simulink model "ISTR_Discrete_Non_Linear"  (Simulink 9.1)
settings: Solver=ode45  StartTime=0.0  StopTime=15*Tuc  RelTol=1e-3  EnableMultiTasking=on
values from neighbouring files (symbols this model uses):
  a0 = 0    [ISTR_Discrete_Non_Linear_init.m]
  a1 = -1.991    [ISTR_Discrete_Non_Linear_init.m]
  a2 = 0.9968    [ISTR_Discrete_Non_Linear_init.m]
  A_ch1 = pi*(100/2)^2    (= 7853.98163397)    [ISTR_Discrete_Non_Linear_init.m]
  A_ch2 = A_ch1    (= 7853.98163397)    [ISTR_Discrete_Non_Linear_init.m]
  A_p = pi*(d/2)^2    (= 78.5398163397)    [ISTR_Discrete_Non_Linear_init.m]
  am1 = -1.888    [ISTR_Discrete_Non_Linear_init.m]
  am2 = 0.894    [ISTR_Discrete_Non_Linear_init.m]
  b = 0.21    [ISTR_Discrete_Non_Linear_init.m]
  b0 = 1.247    [ISTR_Discrete_Non_Linear_init.m]
  b1 = 1.245    [ISTR_Discrete_Non_Linear_init.m]
  bm0 = 1+am1+am2    (= 0.006)    [ISTR_Discrete_Non_Linear_init.m]
  C = 0.45*10^-3    (= 0.00045)    [ISTR_Discrete_Non_Linear_init.m]
  d = 10    [ISTR_Discrete_Non_Linear_init.m]
  Gamma = 1.41    [ISTR_Discrete_Non_Linear_init.m]
  h0_1 = 150    [ISTR_Discrete_Non_Linear_init.m]
  h0_2 = h0_1    (= 150)    [ISTR_Discrete_Non_Linear_init.m]
  h1_init = h0_1/2    (= 75)    [ISTR_Discrete_Non_Linear_init.m]
  h2_init = h0_2/2    (= 75)    [ISTR_Discrete_Non_Linear_init.m]
  l = 1000    [ISTR_Discrete_Non_Linear_init.m]
  lambda = 0.95    [ISTR_Discrete_Non_Linear_init.m]
  mu = 10^-3*10^-5    (= 1e-08)    [ISTR_Discrete_Non_Linear_init.m]
  P2_init = 1.0    (= 1)    [ISTR_Discrete_Non_Linear_init.m]
  P_atm = 1    [ISTR_Discrete_Non_Linear_init.m]
  P_init = 1*eye(4,4)    [ISTR_Discrete_Non_Linear_init.m]
  Ps = 1.2    [ISTR_Discrete_Non_Linear_init.m]
  Q_amp = 30    [ISTR_Discrete_Non_Linear_init.m]
  R = 287*10^4    (= 2870000)    [ISTR_Discrete_Non_Linear_init.m]
  Roh_air = 1.2    [ISTR_Discrete_Non_Linear_init.m]
  Roh_w = 998    [ISTR_Discrete_Non_Linear_init.m]
  T0 = 273+20    (= 293)    [ISTR_Discrete_Non_Linear_init.m]
  T1 = 273+20    (= 293)    [ISTR_Discrete_Non_Linear_init.m]
  T2 = T1    (= 293)    [ISTR_Discrete_Non_Linear_init.m]
  Tf = 273+20    (= 293)    [ISTR_Discrete_Non_Linear_init.m]
  theta_init = theta_linear    [ISTR_Discrete_Non_Linear_init.m]
  Ts = 273+20    (= 293)    [ISTR_Discrete_Non_Linear_init.m]
  Tsamp = 1/100    (= 0.01)    [ISTR_Discrete_Non_Linear_init.m]
  Tuc = 3    [ISTR_Discrete_Non_Linear_init.m]
  Wn = 8    [ISTR_Discrete_Non_Linear_init.m]
  zetta = 0.7    [ISTR_Discrete_Non_Linear_init.m]
libraries: commnoisgen2 x1
settings Model: Creator=gshaver  LastModifiedBy=Ahmad
settings DataIOCC: LimitDataPoints=on  SignalLoggingSaveFormat=ModelDataLogs
settings OptimizationCC: ExpressionDepthLimit=2147483647
settings DebuggingCC: SolverPrmCheckMsg=warning  FcnCallInpInsideContextMsg=warning  StateNameClashWarn=warning
settings GRTTargetCC: GeneratePreprocessorConditionals=Disable all

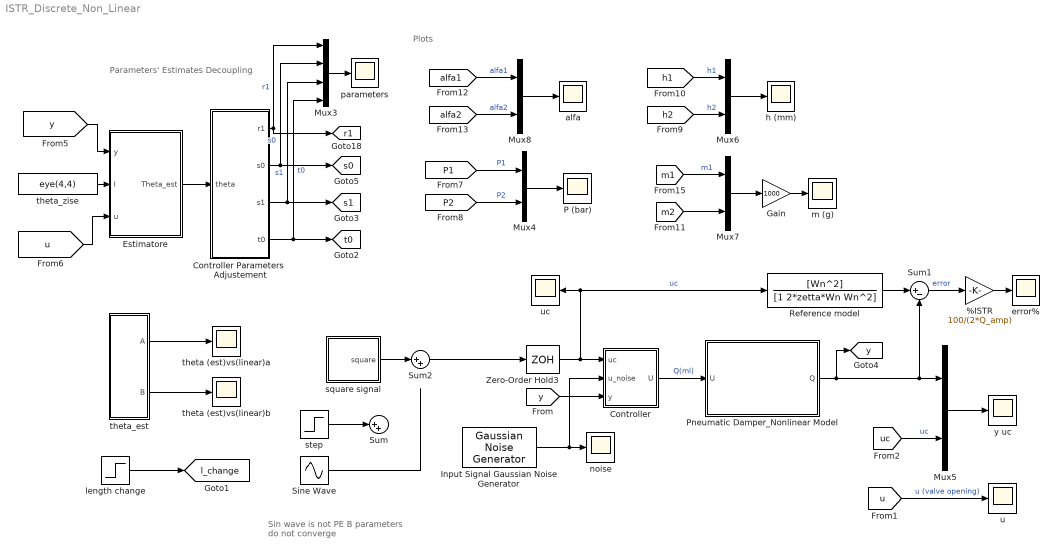
== system ISTR_Discrete_Non_Linear ==
  note: Plots
  note: Sin wave is not PE
      | B parameters do not converge
  note: Parameters' Estimates Decoupling
  %ISTR : Gain  Gain=100/(2*Q_amp)
  Controller : Subsystem
  Controller Parameters  Adjustement : Subsystem
  Estimatore : Subsystem
  Gain : Gain  Gain=1000
  Input Signal Gaussian Noise Generator : commnoisgen2/Gaussian Noise Generator  m=0  d=Noise  s=41  Ts=1/100  frameBased=off  sampPerFrame=1  orient=off  outDataType=double
  Mux3 : Mux
  Mux{4..8} (5 alike) : Mux  Inputs=2
  P (bar) : Scope
  Pneumatic Damper_Nonlinear Model : Subsystem
  Reference model : TransferFcn  Numerator=[Wn^2]  Denominator=[1 2*zetta*Wn Wn^2]
  Sine Wave : Sin  Amplitude=10  Frequency=Tuc  SampleTime=0
  Sum : Sum  Inputs=|++
  Sum1 : Sum  Inputs=|+-
  Sum2 : Sum  Inputs=|++
  Zero-Order Hold3 : ZeroOrderHold  SampleTime=Tsamp
  alfa : Scope
  error% : Scope
  h (mm) : Scope
  length change : Step  Time=0  After=0  SampleTime=0
  m (g) : Scope
  noise : Scope
  parameters : Scope
  square signal : Subsystem
  step : Step  Time=0.01  Before=10  After=0  SampleTime=0
  theta (est)vs(linear)a : Scope
  theta (est)vs(linear)b : Scope
  theta_est : Subsystem
  theta_zise : Constant  Value=eye(4,4)  VectorParams1D=off
  u : Scope
  uc : Scope
  y uc : Scope
  tag scope: l_change=global, r1=global, s0=global, s1=global, t0=global, y=global
  wires:
  [y] -> Estimatore/1(y)
  theta_zise/1 -> Estimatore/2(I)
  [u] -> Estimatore/3(u)
  step/1 -> Sum/1
  Controller Parameters  Adjustement/4("t0 ") -> Mux3/4, [t0]  "t0"
  Controller Parameters  Adjustement/1("r1 ") -> Mux3/1, [r1]  "r1"
  Controller Parameters  Adjustement/2("s0 ") -> Mux3/2, [s0]  "s0"
  Controller Parameters  Adjustement/3("s1 ") -> Mux3/3, [s1]  "s1"
  Sine Wave/1 -> ?
  Controller/1(U) -> Pneumatic Damper_Nonlinear Model/1(U)  "Q(ml)"
  Mux5/1 -> y uc/1
  [u] -> u/1  "u (valve opening)"
  [uc] -> Mux5/2  "uc"
  Estimatore/1(Theta_est) -> Controller Parameters  Adjustement/1(theta)
  Sum1/1 -> %ISTR/1  "error"
  Zero-Order Hold3/1 -> Controller/1(uc), uc/1, Reference model/1  "uc"
  Input Signal Gaussian Noise Generator/1 -> Controller/2(u_noise), noise/1
  length change/1 -> [l_change]
  Mux3/1 -> parameters/1
  [P1] -> Mux4/1  "P1"
  [P2] -> Mux4/2  "P2"
  Mux4/1 -> P (bar)/1
  [h1] -> Mux6/1  "h1"
  [h2] -> Mux6/2  "h2"
  Mux6/1 -> h (mm)/1
  [m1] -> Mux7/1  "m1"
  [m2] -> Mux7/2
  Mux7/1 -> Gain/1
  Gain/1 -> m (g)/1
  [alfa1] -> Mux8/1  "alfa1"
  [alfa2] -> Mux8/2  "alfa2"
  Mux8/1 -> alfa/1
  Reference model/1 -> Sum1/1
  square signal/1(square) -> Sum2/1
  theta_est/1(A) -> theta (est)vs(linear)a/1
  theta_est/2(B) -> theta (est)vs(linear)b/1
  %ISTR/1 -> error%/1
  Sum2/1 -> Zero-Order Hold3/1
  Pneumatic Damper_Nonlinear Model/1("Q  ") -> [y], Mux5/1, Sum1/2
  [y] -> Controller/3(y)

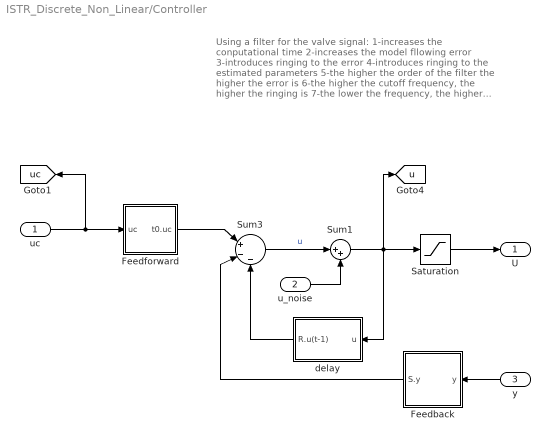
== system ISTR_Discrete_Non_Linear/Controller ==
  note: Using a filter for the valve signal:
      | 1-increases the conputational time
      | 2-increases the model fllowing error
      | 3-introduces ringing to the error
      | 4-introduces ringing to the estimated parameters
      | 5-the higher the order of the filter the higher the error is
      | 6-the higher the cutoff frequency, the higher the ringing is
      | 7-the lower the frequency, the higher the error is
  uc : Inport
  u_noise : Inport  Port=2
  y : Inport  Port=3
  Feedback : Subsystem
  Feedforward : Subsystem
  Saturation : Saturate  UpperLimit=1  LowerLimit=-1
  Sum1 : Sum  Inputs=|++
  Sum3 : Sum  Inputs=|+--
  delay : Subsystem
  U : Outport
  tag scope: u=global, uc=global
  wires:
  uc/1 -> Feedforward/1(uc), [uc]
  Feedforward/1(t0.uc) -> Sum3/1
  Feedback/1(S.y) -> Sum3/2
  delay/1(R.u(t-1)) -> Sum3/3
  Sum3/1 -> Sum1/1  "u"
  u_noise/1 -> Sum1/2
  Sum1/1 -> Saturation/1, [u], delay/1(u)
  Saturation/1 -> U/1
  y/1 -> Feedback/1(y)

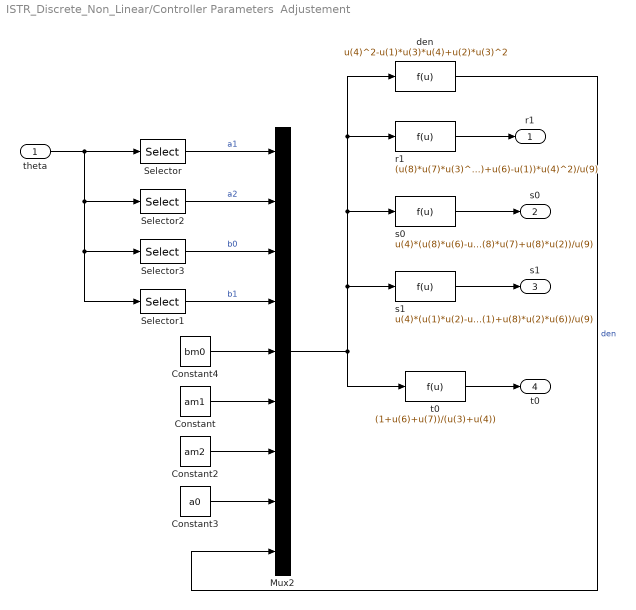
== system ISTR_Discrete_Non_Linear/Controller Parameters  Adjustement ==
  theta : Inport
  Constant : Constant  Value=am1
  Constant2 : Constant  Value=am2
  Constant3 : Constant  Value=a0
  Constant4 : Constant  Value=bm0
  Mux2 : Mux  Inputs=9
  Selector : Selector  NumberOfDimensions=2  InputPortWidth=3  IndexOptions=Index vector (dialog),Index vector (dialog)  Indices=1,1  OutputSizes=1,1
  Selector1 : Selector  NumberOfDimensions=2  InputPortWidth=3  IndexOptions=Index vector (dialog),Index vector (dialog)  Indices=4,1  OutputSizes=1,1
  Selector2 : Selector  NumberOfDimensions=2  InputPortWidth=3  IndexOptions=Index vector (dialog),Index vector (dialog)  Indices=2,1  OutputSizes=1,1
  Selector3 : Selector  NumberOfDimensions=2  InputPortWidth=3  IndexOptions=Index vector (dialog),Index vector (dialog)  Indices=3,1  OutputSizes=1,1
  den : Fcn  Expr=u(4)^2-u(1)*u(3)*u(4)+u(2)*u(3)^2
  r1 : Fcn  Expr=(u(8)*u(7)*u(3)^2+(u(2)-u(7)-u(8)*u(6))*u(3)*u(4)+(u(8)+u(6)-u(1))*u(4)^2)/u(9)
  s0 : Fcn  Expr=u(4)*(u(8)*u(6)-u(2)-u(6)*u(1)+u(1)^2+u(7)-u(1)*u(8))/u(9)+u(3)*(u(6)*u(2)-u(1)*u(2)-u(8)*u(7)+u(8)*u(2))/u(9)
  s1 : Fcn  Expr=u(4)*(u(1)*u(2)-u(6)*u(2)+u(8)*u(7)-u(8)*u(2))/u(9)+u(3)*(u(2)*u(7)-u(2)^2-u(8)*u(7)*u(1)+u(8)*u(2)*u(6))/u(9)
  t0 : Fcn  Expr=(1+u(6)+u(7))/(u(3)+u(4))
  "r1 " : Outport
  "s0 " : Outport  Port=2
  "s1 " : Outport  Port=3
  "t0 " : Outport  Port=4
  wires:
  t0/1 -> "t0 "/1
  s1/1 -> "s1 "/1
  r1/1 -> "r1 "/1
  Mux2/1 -> den/1, r1/1, s0/1, s1/1, t0/1
  s0/1 -> "s0 "/1
  Constant/1 -> Mux2/6
  Selector/1 -> Mux2/1  "a1"
  Constant4/1 -> Mux2/5
  Constant2/1 -> Mux2/7
  Constant3/1 -> Mux2/8
  den/1 -> Mux2/9  "den"
  Selector3/1 -> Mux2/3  "b0"
  theta/1 -> Selector1/1, Selector3/1, Selector2/1, Selector/1
  Selector1/1 -> Mux2/4  "b1"
  Selector2/1 -> Mux2/2  "a2"

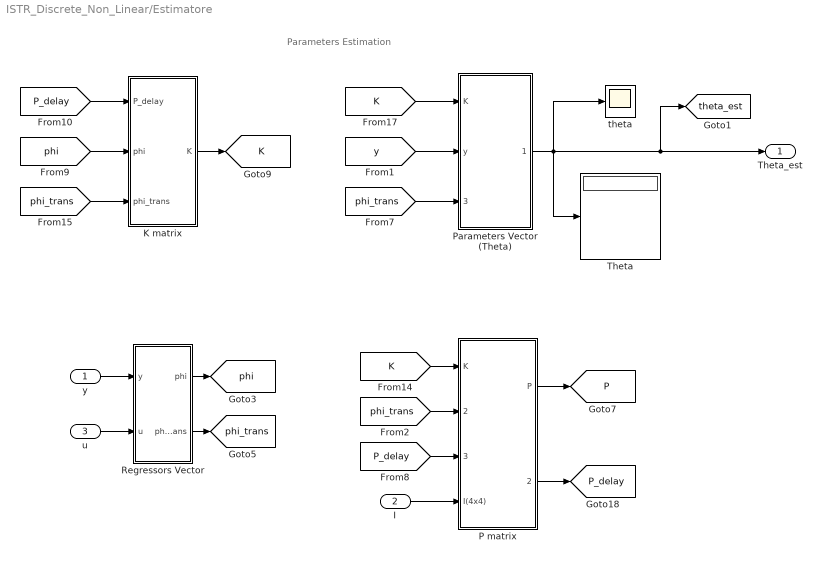
== system ISTR_Discrete_Non_Linear/Estimatore ==
  note: Parameters Estimation
  y : Inport
  I : Inport  Port=2
  u : Inport  Port=3
  K matrix : Subsystem
  P matrix : Subsystem
  Parameters Vector (Theta) : Subsystem
  Regressors Vector : Subsystem
  Theta : Display
  theta : Scope
  Theta_est : Outport
  tag scope: K=global, P=global, P_delay=global, phi=global, phi_trans=global, theta_est=global
  wires:
  [K] -> Parameters Vector (Theta)/1(K)
  y/1 -> Regressors Vector/1(y)
  [phi_trans] -> K matrix/3(phi_trans)
  [phi] -> K matrix/2(phi)
  [P_delay] -> K matrix/1(P_delay)
  K matrix/1(K) -> [K]
  [phi_trans] -> Parameters Vector (Theta)/3(phi_trans)
  Regressors Vector/2(phi_trans) -> [phi_trans]
  u/1 -> Regressors Vector/2(u)
  Regressors Vector/1(phi) -> [phi]
  I/1 -> P matrix/4(I(4x4))
  P matrix/2("P_delay ") -> [P_delay]
  [K] -> P matrix/1(K)
  [phi_trans] -> P matrix/2(phi_trans)
  [P_delay] -> P matrix/3(P_delay)
  P matrix/1(P) -> [P]
  Parameters Vector (Theta)/1(Theta_est) -> theta/1, [theta_est], Theta_est/1, Theta/1
  [y] -> Parameters Vector (Theta)/2(y)

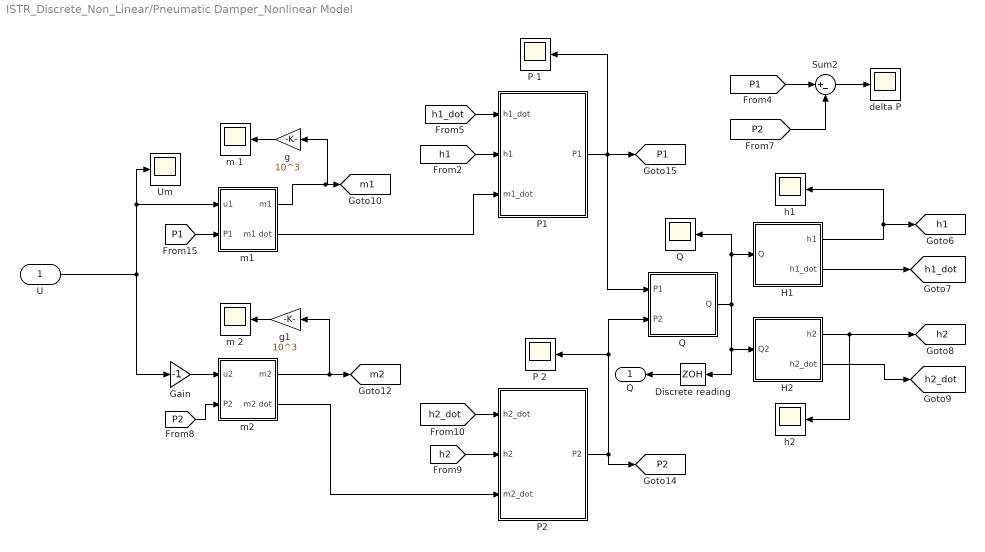
== system ISTR_Discrete_Non_Linear/Pneumatic Damper_Nonlinear Model ==
  U : Inport
  Discrete reading : ZeroOrderHold  SampleTime=Tsamp
  Gain : Gain  Gain=-1
  H1 : Subsystem
  H2 : Subsystem
  P 1 : Scope
  P 2 : Scope
  P1 : Subsystem
  P2 : Subsystem
  Q : Subsystem
  "Q " : Scope
  Sum2 : Sum  Inputs=|+-
  Um : Scope
  delta P : Scope
  g : Gain  Gain=10^3
  g1 : Gain  Gain=10^3
  h1 : Scope
  h2 : Scope
  m 1 : Scope
  m 2 : Scope
  m1 : Subsystem
  m2 : Subsystem
  "Q  " : Outport
  tag scope: P1=global, P2=global, h1=global, h1_dot=global, h2=global, h2_dot=global, m1=global, m2=global
  wires:
  H1/1(h1) -> [h1], h1/1
  H1/2(h1_dot) -> [h1_dot]
  H2/2(h2_dot) -> [h2_dot]
  H2/1(h2) -> h2/1, [h2]
  m1/1(m1) -> g/1, [m1]
  m2/1(m2) -> g1/1, [m2]
  m2/2(m2 dot) -> P2/3(m2_dot)
  [h2_dot] -> P2/1(h2_dot)
  [h1] -> P1/2(h1)
  [h2] -> P2/2(h2)
  P2/1(P2) -> [P2], P 2/1, Q/2(P2)
  U/1 -> Um/1, m1/1(u1), Gain/1
  P1/1(P1) -> P 1/1, Q/1(P1), [P1]
  Gain/1 -> m2/1(u2)
  Q/1(Q) -> Discrete reading/1, H2/1(Q2), H1/1(Q), "Q "/1
  [h1_dot] -> P1/1(h1_dot)
  g/1 -> m 1/1
  [P1] -> Sum2/1
  Sum2/1 -> delta P/1
  [P2] -> Sum2/2
  m1/2(m1 dot) -> P1/3(m1_dot)
  [P2] -> m2/2(P2)
  g1/1 -> m 2/1
  [P1] -> m1/2(P1)
  Discrete reading/1 -> "Q  "/1

== system ISTR_Discrete_Non_Linear/square signal ==
  Pulse Generator1 : DiscretePulseGenerator  PulseType=Time based  Amplitude=-Q_amp  Period=Tuc  PulseWidth=50  PhaseDelay=Tuc/2
  Pulse Generator3 : DiscretePulseGenerator  PulseType=Time based  Amplitude=Q_amp  Period=Tuc  PulseWidth=50
  Sum3 : Sum  Inputs=|++
  square : Outport
  wires:
  Pulse Generator3/1 -> Sum3/1
  Sum3/1 -> square/1
  Pulse Generator1/1 -> Sum3/2

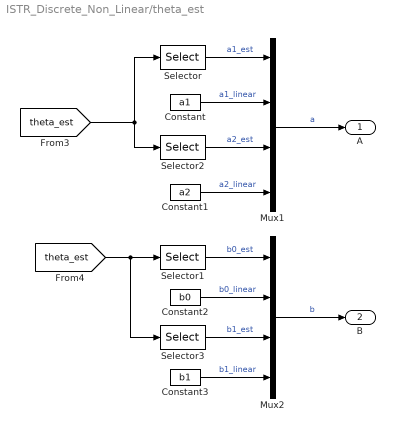
== system ISTR_Discrete_Non_Linear/theta_est ==
  Constant : Constant  Value=a1
  Constant1 : Constant  Value=a2
  Constant2 : Constant  Value=b0
  Constant3 : Constant  Value=b1
  Mux1 : Mux
  Mux2 : Mux
  Selector : Selector  NumberOfDimensions=2  InputPortWidth=3  IndexOptions=Index vector (dialog),Index vector (dialog)  Indices=1,1  OutputSizes=1,1
  Selector1 : Selector  NumberOfDimensions=2  InputPortWidth=3  IndexOptions=Index vector (dialog),Index vector (dialog)  Indices=3,1  OutputSizes=1,1
  Selector2 : Selector  NumberOfDimensions=2  InputPortWidth=3  IndexOptions=Index vector (dialog),Index vector (dialog)  Indices=2,1  OutputSizes=1,1
  Selector3 : Selector  NumberOfDimensions=2  InputPortWidth=3  IndexOptions=Index vector (dialog),Index vector (dialog)  Indices=4,1  OutputSizes=1,1
  A : Outport
  B : Outport  Port=2
  wires:
  Selector2/1 -> Mux1/3  "a2_est"
  Constant3/1 -> Mux2/4  "b1_linear"
  Constant1/1 -> Mux1/4  "a2_linear"
  [theta_est] -> Selector/1, Selector2/1
  Constant2/1 -> Mux2/2  "b0_linear"
  Constant/1 -> Mux1/2  "a1_linear"
  Selector3/1 -> Mux2/3  "b1_est"
  Mux2/1 -> B/1  "b"
  [theta_est] -> Selector1/1, Selector3/1
  Selector/1 -> Mux1/1  "a1_est"
  Mux1/1 -> A/1  "a"
  Selector1/1 -> Mux2/1  "b0_est"

== system ISTR_Discrete_Non_Linear/Controller/Feedback ==
  y : Inport
  Product1 : Product
  Product3 : Product
  Sum4 : Sum  Inputs=|++
  Unit Delay : UnitDelay  SampleTime=-1
  S.y : Outport
  wires:
  y/1 -> Product3/2, Unit Delay/1
  Sum4/1 -> S.y/1
  Product1/1 -> Sum4/2
  Unit Delay/1 -> Product1/1  "y(t-1)"
  Product3/1 -> Sum4/1
  [s1] -> Product1/2
  [s0] -> Product3/1

== system ISTR_Discrete_Non_Linear/Controller/Feedforward ==
  uc : Inport
  Product2 : Product
  t0.uc : Outport
  wires:
  Product2/1 -> t0.uc/1
  [t0] -> Product2/2
  uc/1 -> Product2/1

== system ISTR_Discrete_Non_Linear/Controller/delay ==
  u : Inport
  Product4 : Product
  Unit Delay1 : UnitDelay  SampleTime=-1
  R.u(t-1) : Outport
  wires:
  u/1 -> Unit Delay1/1
  Unit Delay1/1 -> Product4/2  "u(t-1)"
  Product4/1 -> R.u(t-1)/1
  [r1] -> Product4/1

== system ISTR_Discrete_Non_Linear/Estimatore/K matrix ==
  P_delay : Inport
  phi : Inport  Port=2
  phi_trans : Inport  Port=3
  Lambda2 : Constant  Value=lambda  VectorParams1D=off
  Matrix Multiply2 : Product  Multiplication=Matrix(*)
  Matrix Multiply6 : Product  Inputs=***  Multiplication=Matrix(*)
  Matrix Multiply7 : Product  Inputs=/  Multiplication=Matrix(*)
  Matrix Multiply9 : Product  Inputs=**  Multiplication=Matrix(*)
  Sum4 : Sum  Inputs=|++
  K : Outport
  wires:
  Matrix Multiply9/1 -> K/1
  Matrix Multiply7/1 -> Matrix Multiply9/2
  Matrix Multiply2/1 -> Matrix Multiply9/1
  P_delay/1 -> Matrix Multiply6/2, Matrix Multiply2/1
  Lambda2/1 -> Sum4/2
  Matrix Multiply6/1 -> Sum4/1
  Sum4/1 -> Matrix Multiply7/1
  phi_trans/1 -> Matrix Multiply6/1
  phi/1 -> Matrix Multiply6/3, Matrix Multiply2/2

== system ISTR_Discrete_Non_Linear/Estimatore/P matrix ==
  K : Inport
  phi_trans : Inport  Port=2
  P_delay : Inport  Port=3
  I(4x4) : Inport  Port=4
  Gain : Gain  Gain=1/lambda
  Matrix Multiply5 : Product  Multiplication=Matrix(*)
  Matrix Multiply8 : Product  Multiplication=Matrix(*)
  Sum5 : Sum  Inputs=|-+
  Unit Delay6 : UnitDelay  InitialCondition=P_init  SampleTime=Tsamp
  P : Outport
  "P_delay " : Outport  Port=2
  wires:
  phi_trans/1 -> Matrix Multiply8/2
  Matrix Multiply8/1 -> Sum5/1
  K/1 -> Matrix Multiply8/1
  Sum5/1 -> Matrix Multiply5/1
  P_delay/1 -> Matrix Multiply5/2
  Matrix Multiply5/1 -> Gain/1
  Gain/1 -> P/1, Unit Delay6/1
  Unit Delay6/1 -> "P_delay "/1
  I(4x4)/1 -> Sum5/2

== system ISTR_Discrete_Non_Linear/Estimatore/Parameters Vector (Theta) ==
  K : Inport
  y : Inport  Port=2
  phi_trans : Inport  Port=3
  K17 : Scope
  Matrix Multiply3 : Product  Multiplication=Matrix(*)
  Matrix Multiply4 : Product  Multiplication=Matrix(*)
  Sum1 : Sum  Inputs=|+-
  Sum3 : Sum  Inputs=|++
  Unit Delay1 : UnitDelay  InitialCondition=theta_init  SampleTime=Tsamp
  Theta_est : Outport
  wires:
  K/1 -> Matrix Multiply4/1, K17/1
  Matrix Multiply3/1 -> Sum1/2
  phi_trans/1 -> Matrix Multiply3/1
  Unit Delay1/1 -> Sum3/2, Matrix Multiply3/2  "theta(t-1)"
  Sum1/1 -> Matrix Multiply4/2  "theta"
  Matrix Multiply4/1 -> Sum3/1
  Sum3/1 -> Theta_est/1, Unit Delay1/1
  y/1 -> Sum1/1

== system ISTR_Discrete_Non_Linear/Estimatore/Regressors Vector ==
  y : Inport
  u : Inport  Port=2
  Gain : Gain  Gain=-1
  Regressors : Scope
  Transpose : Math  Operator=transpose  SaturateOnIntegerOverflow=on
  Unit Delay1 : UnitDelay  SampleTime=Tsamp
  Unit Delay2 : UnitDelay  SampleTime=Tsamp
  Unit Delay3 : UnitDelay  InitialCondition=0.1  SampleTime=Tsamp
  Unit Delay6 : UnitDelay  SampleTime=Tsamp
  Vector Concatenate : Concatenate  NumInputs=4  Mode=Multidimensional array
  phi : Outport
  phi_trans : Outport  Port=2
  wires:
  Gain/1 -> Unit Delay1/1
  u/1 -> Unit Delay6/1
  Vector Concatenate/1 -> phi/1, Regressors/1, Transpose/1
  y/1 -> Gain/1
  Unit Delay2/1 -> Vector Concatenate/2
  Transpose/1 -> phi_trans/1
  Unit Delay3/1 -> Vector Concatenate/4
  Unit Delay1/1 -> Unit Delay2/1, Vector Concatenate/1
  Unit Delay6/1 -> Vector Concatenate/3, Unit Delay3/1

== system ISTR_Discrete_Non_Linear/Pneumatic Damper_Nonlinear Model/H1 ==
  Q : Inport
  Constant : Constant  Value=A_ch1
  Divide : Product  Inputs=*/
  Integrator : Integrator  InitialCondition=h1_init
  cm-mm : Gain  Gain=-10^3
  h1 : Outport
  h1_dot : Outport  Port=2
  wires:
  Q/1 -> Divide/1
  Integrator/1 -> h1/1  "h1"
  cm-mm/1 -> h1_dot/1, Integrator/1  "h1_dot"
  Divide/1 -> cm-mm/1
  Constant/1 -> Divide/2

== system ISTR_Discrete_Non_Linear/Pneumatic Damper_Nonlinear Model/H2 ==
  Q2 : Inport
  A_pressure_chamber2 : Constant  Value=A_ch2
  Divide : Product  Inputs=*/
  Integrator : Integrator  InitialCondition=h2_init
  cm-mm : Gain  Gain=10^3
  h2 : Outport
  h2_dot : Outport  Port=2
  wires:
  A_pressure_chamber2/1 -> Divide/2
  Q2/1 -> Divide/1
  Integrator/1 -> h2/1  "h2"
  Divide/1 -> cm-mm/1  "h2_dot"
  cm-mm/1 -> Integrator/1, h2_dot/1

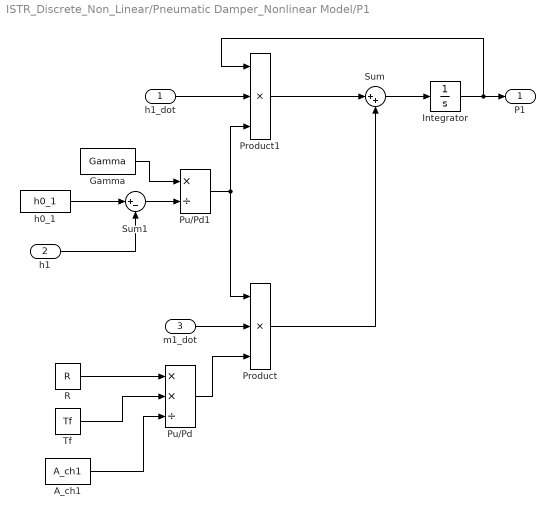
== system ISTR_Discrete_Non_Linear/Pneumatic Damper_Nonlinear Model/P1 ==
  h1_dot : Inport
  h1 : Inport  Port=2
  m1_dot : Inport  Port=3
  A_ch1 : Constant  Value=A_ch1
  Gamma : Constant  Value=Gamma
  Integrator : Integrator  InitialCondition=P2_init
  Product : Product  Inputs=3
  Product1 : Product  Inputs=3
  Pu/Pd : Product  Inputs=**/
  Pu/Pd1 : Product  Inputs=*/
  R : Constant  Value=R
  Sum : Sum  Inputs=|++
  Sum1 : Sum  Inputs=|+-
  Tf : Constant  Value=Tf
  h0_1 : Constant  Value=h0_1
  P1 : Outport
  wires:
  R/1 -> Pu/Pd/1
  A_ch1/1 -> Pu/Pd/3
  Gamma/1 -> Pu/Pd1/1
  Sum1/1 -> Pu/Pd1/2
  h0_1/1 -> Sum1/1
  Tf/1 -> Pu/Pd/2
  Pu/Pd1/1 -> Product/1, Product1/3
  Pu/Pd/1 -> Product/3
  Sum/1 -> Integrator/1
  Integrator/1 -> Product1/1, P1/1
  Product1/1 -> Sum/1
  Product/1 -> Sum/2
  h1_dot/1 -> Product1/2
  h1/1 -> Sum1/2
  m1_dot/1 -> Product/2

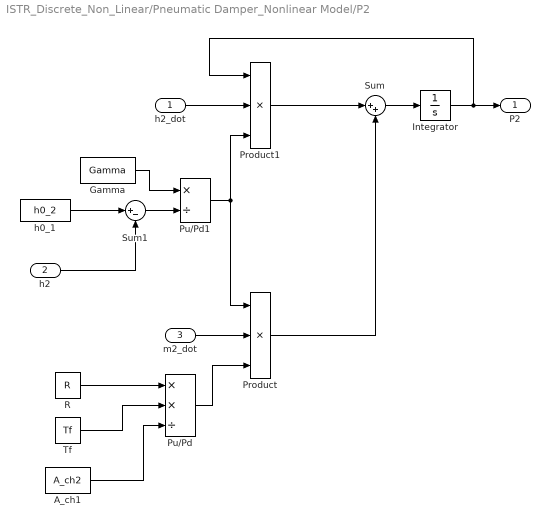
== system ISTR_Discrete_Non_Linear/Pneumatic Damper_Nonlinear Model/P2 ==
  h2_dot : Inport
  h2 : Inport  Port=2
  m2_dot : Inport  Port=3
  A_ch1 : Constant  Value=A_ch2
  Gamma : Constant  Value=Gamma
  Integrator : Integrator  InitialCondition=P2_init
  Product : Product  Inputs=3
  Product1 : Product  Inputs=3
  Pu/Pd : Product  Inputs=**/
  Pu/Pd1 : Product  Inputs=*/
  R : Constant  Value=R
  Sum : Sum  Inputs=|++
  Sum1 : Sum  Inputs=|+-
  Tf : Constant  Value=Tf
  h0_1 : Constant  Value=h0_2
  P2 : Outport
  wires:
  R/1 -> Pu/Pd/1
  A_ch1/1 -> Pu/Pd/3
  Integrator/1 -> Product1/1, P2/1
  Gamma/1 -> Pu/Pd1/1
  Sum1/1 -> Pu/Pd1/2
  h0_1/1 -> Sum1/1
  Tf/1 -> Pu/Pd/2
  Pu/Pd1/1 -> Product/1, Product1/3
  Pu/Pd/1 -> Product/3
  Sum/1 -> Integrator/1
  Product1/1 -> Sum/1
  Product/1 -> Sum/2
  h2_dot/1 -> Product1/2
  h2/1 -> Sum1/2
  m2_dot/1 -> Product/2

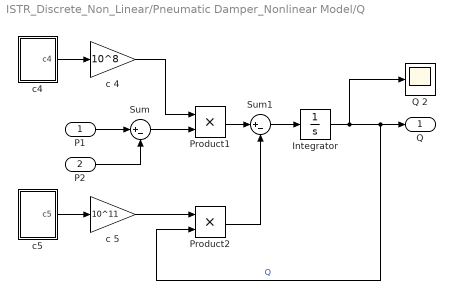
== system ISTR_Discrete_Non_Linear/Pneumatic Damper_Nonlinear Model/Q ==
  P1 : Inport
  P2 : Inport  Port=2
  Integrator : Integrator
  Product1 : Product
  Product2 : Product
  Q 2 : Scope
  Sum : Sum  Inputs=|+-
  Sum1 : Sum  Inputs=|+-
  c 4 : Gain  Gain=10^8
  c 5 : Gain  Gain=10^11
  c4 : Subsystem
  c5 : Subsystem
  Q : Outport
  wires:
  P1/1 -> Sum/1
  P2/1 -> Sum/2
  Sum/1 -> Product1/2
  Product1/1 -> Sum1/1
  Integrator/1 -> Q 2/1, Product2/2, Q/1  "Q"
  Product2/1 -> Sum1/2
  Sum1/1 -> Integrator/1
  c4/1(c4) -> c 4/1
  c 4/1 -> Product1/1
  c 5/1 -> Product2/1
  c5/1(c5) -> c 5/1

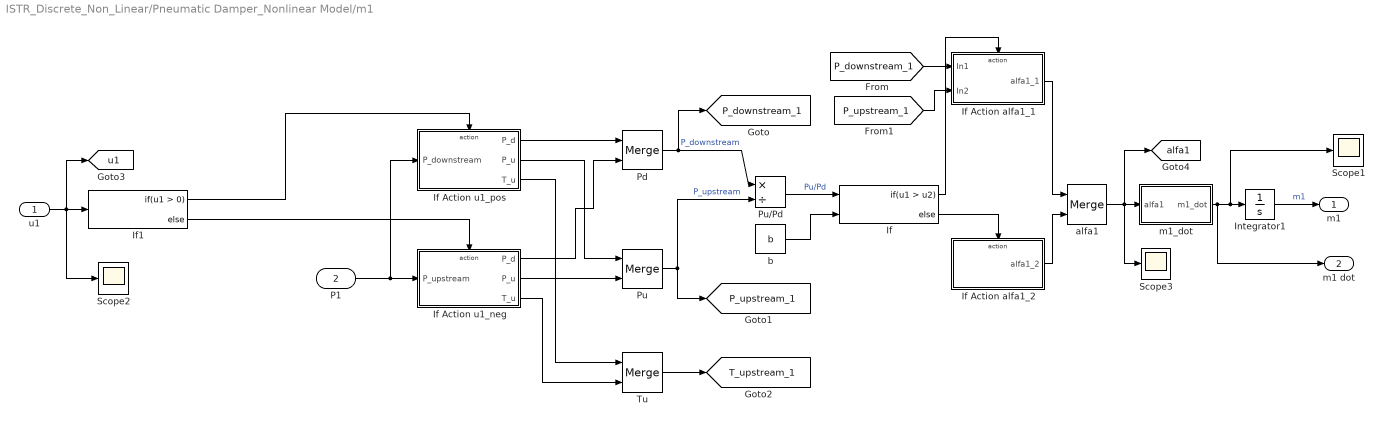
== system ISTR_Discrete_Non_Linear/Pneumatic Damper_Nonlinear Model/m1 ==
  u1 : Inport
  P1 : Inport  Port=2
  If : If  NumInputs=2  IfExpression=u1 > u2
  If Action alfa1_1 : Subsystem  TreatAsAtomicUnit=on
  If Action alfa1_2 : Subsystem  TreatAsAtomicUnit=on
  If Action u1_neg : Subsystem  TreatAsAtomicUnit=on
  If Action u1_pos : Subsystem  TreatAsAtomicUnit=on
  If1 : If
  Integrator1 : Integrator
  Pd : Merge
  Pu : Merge
  Pu/Pd : Product  Inputs=*/
  Scope1 : Scope
  Scope2 : Scope
  Scope3 : Scope
  Tu : Merge
  alfa1 : Merge
  b : Constant  Value=b
  m1_dot : Subsystem
  m1 : Outport
  m1 dot : Outport  Port=2
  tag scope: P_downstream_1=global, P_upstream_1=global, T_upstream_1=global, alfa1=global, u1=global
  wires:
  alfa1/1 -> [alfa1], Scope3/1, m1_dot/1(alfa1)
  Integrator1/1 -> m1/1  "m1"
  If1/2 -> If Action u1_neg/Action
  u1/1 -> Scope2/1, [u1], If1/1
  If1/1 -> If Action u1_pos/Action
  Pu/Pd/1 -> If/1  "Pu/Pd"
  If/1 -> If Action alfa1_1/Action
  If/2 -> If Action alfa1_2/Action
  b/1 -> If/2
  Pd/1 -> Pu/Pd/1, [P_downstream_1]  "P_downstream"
  Pu/1 -> Pu/Pd/2, [P_upstream_1]  "P_upstream"
  If Action u1_pos/1(P_d) -> Pd/1
  If Action alfa1_2/1(alfa1_2) -> alfa1/2
  If Action alfa1_1/1(alfa1_1) -> alfa1/1
  If Action u1_neg/1(P_d) -> Pd/2
  If Action u1_pos/2(P_u) -> Pu/1
  If Action u1_neg/2(P_u) -> Pu/2
  m1_dot/1(m1_dot) -> m1 dot/1, Scope1/1, Integrator1/1
  If Action u1_neg/3(T_u) -> Tu/2
  If Action u1_pos/3(T_u) -> Tu/1
  Tu/1 -> [T_upstream_1]
  [P_downstream_1] -> If Action alfa1_1/1(In1)
  [P_upstream_1] -> If Action alfa1_1/2(In2)
  P1/1 -> If Action u1_pos/1(P_downstream), If Action u1_neg/1(P_upstream)

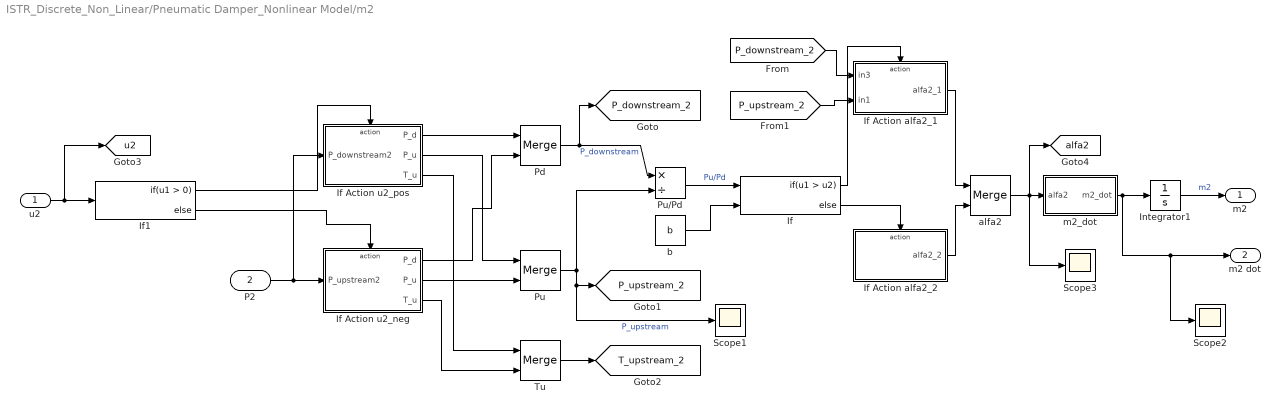
== system ISTR_Discrete_Non_Linear/Pneumatic Damper_Nonlinear Model/m2 ==
  u2 : Inport
  P2 : Inport  Port=2
  If : If  NumInputs=2  IfExpression=u1 > u2
  If Action alfa2_1 : Subsystem  TreatAsAtomicUnit=on
  If Action alfa2_2 : Subsystem  TreatAsAtomicUnit=on
  If Action u2_neg : Subsystem  TreatAsAtomicUnit=on
  If Action u2_pos : Subsystem  TreatAsAtomicUnit=on
  If1 : If
  Integrator1 : Integrator
  Pd : Merge
  Pu : Merge
  Pu/Pd : Product  Inputs=*/
  Scope1 : Scope
  Scope2 : Scope
  Scope3 : Scope
  Tu : Merge
  alfa2 : Merge
  b : Constant  Value=b
  m2_dot : Subsystem
  m2 : Outport
  m2 dot : Outport  Port=2
  tag scope: P_downstream_2=global, P_upstream_2=global, T_upstream_2=global, alfa2=global, u2=global
  wires:
  alfa2/1 -> [alfa2], Scope3/1, m2_dot/1(alfa2)
  Integrator1/1 -> m2/1  "m2"
  If1/2 -> If Action u2_neg/Action
  u2/1 -> [u2], If1/1
  If1/1 -> If Action u2_pos/Action
  Pu/Pd/1 -> If/1  "Pu/Pd"
  If/1 -> If Action alfa2_1/Action
  If/2 -> If Action alfa2_2/Action
  b/1 -> If/2
  Pd/1 -> [P_downstream_2], Pu/Pd/1  "P_downstream"
  Pu/1 -> Pu/Pd/2, Scope1/1, [P_upstream_2]  "P_upstream"
  If Action u2_pos/1(P_d) -> Pd/1
  If Action alfa2_2/1(alfa2_2) -> alfa2/2
  If Action alfa2_1/1(alfa2_1) -> alfa2/1
  If Action u2_neg/1(P_d) -> Pd/2
  If Action u2_pos/2(P_u) -> Pu/1
  If Action u2_neg/2(P_u) -> Pu/2
  m2_dot/1(m2_dot) -> Scope2/1, m2 dot/1, Integrator1/1
  If Action u2_neg/3(T_u) -> Tu/2
  If Action u2_pos/3(T_u) -> Tu/1
  Tu/1 -> [T_upstream_2]
  P2/1 -> If Action u2_neg/1(P_upstream2), If Action u2_pos/1(P_downstream2)
  [P_downstream_2] -> If Action alfa2_1/1(in3)
  [P_upstream_2] -> If Action alfa2_1/2(in1)

== system ISTR_Discrete_Non_Linear/Pneumatic Damper_Nonlinear Model/Q/c4 ==
  Constant1 : Constant  Value=A_p
  Constant2 : Constant  Value=Roh_w
  Constant3 : Constant  Value=l
  Divide1 : Product  Inputs=*//
  Sum : Sum  Inputs=|++
  c4 : Outport
  wires:
  Constant1/1 -> Divide1/1
  Constant2/1 -> Divide1/3
  Constant3/1 -> Sum/1
  Divide1/1 -> c4/1
  Sum/1 -> Divide1/2
  [l_change] -> Sum/2

== system ISTR_Discrete_Non_Linear/Pneumatic Damper_Nonlinear Model/Q/c5 ==
  Constant4 : Constant  Value=mu
  Constant5 : Constant  Value=A_p
  Constant6 : Constant  Value=Roh_w
  Constant7 : Constant  Value=d^4
  Gain1 : Gain  Gain=128/pi
  Pu/Pd : Product  Inputs=**//
  c5 : Outport
  wires:
  Gain1/1 -> c5/1
  Pu/Pd/1 -> Gain1/1
  Constant4/1 -> Pu/Pd/1
  Constant6/1 -> Pu/Pd/3
  Constant5/1 -> Pu/Pd/2
  Constant7/1 -> Pu/Pd/4

== system ISTR_Discrete_Non_Linear/Pneumatic Damper_Nonlinear Model/m1/If Action alfa1_1 ==
  note: Pu
  In1 : Inport
  In2 : Inport  Port=2
  Action Port : ActionPort
  Mux : Mux  Inputs=3
  alfa : Fcn  Expr=sqrt(1-((u(1)/u(2)-u(3))/(1-u(3)))^2)
  b : Constant  Value=b
  alfa1_1 : Outport
  wires:
  b/1 -> Mux/3
  Mux/1 -> alfa/1
  In1/1 -> Mux/1  "Pd"
  In2/1 -> Mux/2
  alfa/1 -> alfa1_1/1

== system ISTR_Discrete_Non_Linear/Pneumatic Damper_Nonlinear Model/m1/If Action alfa1_2 ==
  Action Port : ActionPort
  alfa : Constant
  alfa1_2 : Outport
  wires:
  alfa/1 -> alfa1_2/1

== system ISTR_Discrete_Non_Linear/Pneumatic Damper_Nonlinear Model/m1/If Action u1_neg ==
  P_upstream : Inport
  Action Port : ActionPort
  P_downstream : Constant  Value=P_atm
  T_upstream : Constant  Value=T1
  P_d : Outport
  P_u : Outport  Port=2
  T_u : Outport  Port=3
  wires:
  P_upstream/1 -> P_u/1
  P_downstream/1 -> P_d/1
  T_upstream/1 -> T_u/1

== system ISTR_Discrete_Non_Linear/Pneumatic Damper_Nonlinear Model/m1/If Action u1_pos ==
  P_downstream : Inport
  Action Port : ActionPort
  P_upstream : Constant  Value=Ps
  T_upstream : Constant  Value=Ts
  P_d : Outport
  P_u : Outport  Port=2
  T_u : Outport  Port=3
  wires:
  P_upstream/1 -> P_u/1
  P_downstream/1 -> P_d/1
  T_upstream/1 -> T_u/1

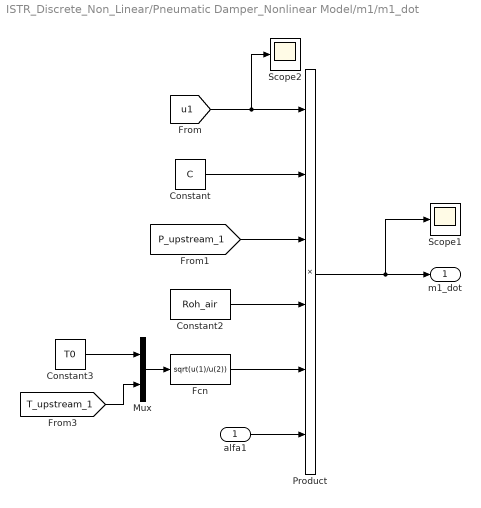
== system ISTR_Discrete_Non_Linear/Pneumatic Damper_Nonlinear Model/m1/m1_dot ==
  alfa1 : Inport
  Constant : Constant  Value=C
  Constant2 : Constant  Value=Roh_air
  Constant3 : Constant  Value=T0
  Fcn : Fcn  Expr=sqrt(u(1)/u(2))
  Mux : Mux  Inputs=2
  Product : Product  Inputs=6
  Scope1 : Scope
  Scope2 : Scope
  m1_dot : Outport
  wires:
  Product/1 -> Scope1/1, m1_dot/1
  [P_upstream_1] -> Product/3
  Constant3/1 -> Mux/1
  alfa1/1 -> Product/6
  Fcn/1 -> Product/5
  Mux/1 -> Fcn/1
  Constant2/1 -> Product/4
  [T_upstream_1] -> Mux/2
  [u1] -> Scope2/1, Product/1
  Constant/1 -> Product/2

== system ISTR_Discrete_Non_Linear/Pneumatic Damper_Nonlinear Model/m2/If Action alfa2_1 ==
  note: Pu
  in3 : Inport
  in1 : Inport  Port=2
  Action Port : ActionPort
  Mux : Mux  Inputs=3
  alfa : Fcn  Expr=sqrt(1-((u(1)/u(2)-u(3))/(1-u(3)))^2)
  b : Constant  Value=b
  alfa2_1 : Outport
  wires:
  b/1 -> Mux/3
  Mux/1 -> alfa/1
  in3/1 -> Mux/1  "Pd"
  in1/1 -> Mux/2
  alfa/1 -> alfa2_1/1

== system ISTR_Discrete_Non_Linear/Pneumatic Damper_Nonlinear Model/m2/If Action alfa2_2 ==
  Action Port : ActionPort
  alfa : Constant
  alfa2_2 : Outport
  wires:
  alfa/1 -> alfa2_2/1

== system ISTR_Discrete_Non_Linear/Pneumatic Damper_Nonlinear Model/m2/If Action u2_neg ==
  P_upstream2 : Inport
  Action Port : ActionPort
  P_downstream2 : Constant  Value=P_atm
  T_upstream2 : Constant  Value=T2
  P_d : Outport
  P_u : Outport  Port=2
  T_u : Outport  Port=3
  wires:
  P_upstream2/1 -> P_u/1
  P_downstream2/1 -> P_d/1
  T_upstream2/1 -> T_u/1

== system ISTR_Discrete_Non_Linear/Pneumatic Damper_Nonlinear Model/m2/If Action u2_pos ==
  P_downstream2 : Inport
  Action Port : ActionPort
  P_upstream2 : Constant  Value=Ps
  T_upstream : Constant  Value=Ts
  P_d : Outport
  P_u : Outport  Port=2
  T_u : Outport  Port=3
  wires:
  P_upstream2/1 -> P_u/1
  P_downstream2/1 -> P_d/1
  T_upstream/1 -> T_u/1

== system ISTR_Discrete_Non_Linear/Pneumatic Damper_Nonlinear Model/m2/m2_dot ==
  alfa2 : Inport
  Constant : Constant  Value=C
  Constant2 : Constant  Value=Roh_air
  Constant3 : Constant  Value=T0
  Fcn : Fcn  Expr=sqrt(u(1)/u(2))
  Mux : Mux  Inputs=2
  Product : Product  Inputs=6
  m2_dot : Outport
  wires:
  Product/1 -> m2_dot/1
  [P_upstream_2] -> Product/3
  Constant3/1 -> Mux/1
  alfa2/1 -> Product/6
  Fcn/1 -> Product/5
  Mux/1 -> Fcn/1
  Constant2/1 -> Product/4
  [T_upstream_2] -> Mux/2
  [u2] -> Product/1
  Constant/1 -> Product/2
